simulink library "ddm"  (R2021b)
settings: Solver=VariableStepAuto  StartTime=0.0  StopTime=10.0  RelTol=1e-3
undefined symbols (not defined in the file or in its folder): ENUM_ADASACCSTA_ERROR, ENUM_ADASACCSTA_OFF, ENUM_ADASACCSTA_STANDBY, ENUM_ADASISASTA_OFF, ENUM_ALLOWMOV_ALLOWREADY, ENUM_APS, ENUM_BRKSTA_ERROR, ENUM_BRKSTA_OFF, ENUM_BRKSTA_ON, ENUM_BRKSW_INVALID, ENUM_BRKSW_OFF, ENUM_BRKSW_ON, ENUM_CHGPREACTERRSTA_OBCPRE, ENUM_DCDCFAULTSTA_ANYFAULTLV1, ENUM_DCDCFAULTSTA_ANYFAULTLV2, ENUM_DRIVETRAIN_AWD, ENUM_DRIVETRAIN_FWD, ENUM_DRIVETRAIN_RWD, ENUM_DRSEATSTA_INVALID, ENUM_EDUDRTSTA_NORMAL, ENUM_EPBSTA_APPLIED, ENUM_EPBSTA_RELEASED, ENUM_HVBATTREADYPRE_READY, ENUM_MCUWARN_LV0, ENUM_MCUWARN_LV1, ENUM_MCUWARN_LV2, ENUM_MCUWARN_LV3, ENUM_MCUWARN_NOERROR, ENUM_OBCFAULTSTA_ANYFAULT, ENUM_PAS_R2F2, ENUM_PDFAULT_BATTPDFAIL, ENUM_PDFAULT_DCDCDISABLE, ENUM_PDFAULT_MCUDISABLE, ENUM_PDFAULT_MCUDISCHRG, ENUM_POWERSTA_OFF, ENUM_POWERSTA_ON, ENUM_POWERSTA_READY, ENUM_POWERSTA_STANDBY, ENUM_PRESSINDI_LOW, ENUM_PUFAULT_BATTUPFAIL, ENUM_PUFAULT_DCDCENABLEFAIL, ENUM_PUFAULT_PRECHRGCHKFAIL, ENUM_PUFAULT_SAFETYCHKFAIL, ENUM_PUSTATE_COMPLETED, ENUM_PWRSTASW_OFF, ENUM_PWRSTASW_OFFA, ENUM_PWRSTASW_OFFCHVCHRG, ENUM_PWRSTASW_OFFCLVCHRG, ENUM_PWRSTASW_ON, ENUM_PWRSTASW_ONHVCHRG, ENUM_PWRSTASW_READY, ENUM_PWRSTASW_STANDBY, ENUM_RANGESTA_12IN, ENUM_SHIFTCOMMAND_D, ENUM_SHIFTCOMMAND_N, ENUM_SHIFTCOMMAND_P, ENUM_SHIFTCOMMAND_R, ENUM_VEHMALFUNLV_2ND, ENUM_VEHMALFUNLV_3RD, ENUM_VEHMALFUNLV_4TH ... (+835)
libraries: hcu_lib x750, $bdroot x12, simulink x5
(part 17 of 28)

== system ddm/DDM/DDM/PMM/Comm err/The CAN signal between VCU and CCU2 is incomplete ==
  note: Diagnostics and Fault Handling
  note: Test Detection Criteria
  note: Fail Safe After Decision
  note: Release Condition After Failure Decision
  note: Release Condition During Failure Detection
  note: Fail Safe During Detection
  note: Test Pass Criteria
  task_time_s : Inport
  VPMM_PowerSta_enum : Inport  Port=2
  VPMM_PwrStaSW_enum : Inport  Port=3
  VDDM_C3CCU2CSChk_flg : Inport  Port=4
  VDDM_C3CCU2LCCFS_flg : Inport  Port=5
  No_CAN3_BUS_OFF : Inport  Port=6
  DTC_clear_request : Inport  Port=7
  Constant15 : Constant  Value=KDDM_C3CCU2CSCFSSW_flg
  Constant{3,16,22,24} (4 alike) : Constant  Value=TRUE
  Constant18 : Constant  Value=KDDM_C3CCU2CSPassTO_s
  Constant19 : Constant  Value=KDDM_C3CCU2CSPassTO_s
  Constant{2,21,23,25,27} (5 alike) : Constant  Value=FALSE
  Constant20 : Constant  Value=KDDM_C3CCU2CSDFSSW_flg
  Constant26 : Constant  Value=ENUM_PWRSTASW_OFF
  Constant28 : Constant  Value=ENUM_PWRSTASW_OFF
  Constant4 : Constant  Value=ENUM_POWERSTA_OFF
  Constant40 : Constant  Value=KDDM_C3CCU2CSDTC_cnt
  Constant41 : Constant  Value=KDDM_C3CCU2CSDetTO_s
  Constant46 : Constant  Value=KDDM_C3CCU2CSDetSW_flg
  Constant48 : Constant  Value=KDDM_C3CCU2CSDTC_cnt
  Constant5 : Constant  Value=KDDM_C3CCU2CSPassSW_flg
  DTC_Couter : hcu_lib/Basic_Blocks/DTC_Couter
  DTC_Info : hcu_lib/Basic_Blocks/DTC_Info
  Data Type Conversion1 : DataTypeConversion  OutDataTypeStr=uint8
  Demux : Demux  Commented=on  Outputs=5
  Equal : RelationalOperator  Operator=~=  OutDataTypeStr=boolean  RndMeth=Simplest
  Equal2 : RelationalOperator  Operator=~=  OutDataTypeStr=boolean  RndMeth=Simplest
  Equal3 : RelationalOperator  OutDataTypeStr=boolean  RndMeth=Simplest
  Equal4 : RelationalOperator  Operator===  OutDataTypeStr=boolean  RndMeth=Simplest
  From19 : From  Commented=on  GotoTag=VDDM_C3CCU2CSDFS_flg
  Goto19 : Goto  Commented=on  GotoTag=VDDM_EDriveSysErrVCUErr_flg
  Logical Operator{1,4,6,9} (4 alike) : Logic  Operator=NOT  AllPortsSameDT=off  OutDataTypeStr=boolean
  Logical Operator12 : Logic  AllPortsSameDT=off  OutDataTypeStr=boolean
  Logical Operator15 : Logic  AllPortsSameDT=off  OutDataTypeStr=boolean
  Logical Operator18 : Logic  AllPortsSameDT=off  OutDataTypeStr=boolean
  Logical Operator19 : Logic  Inputs=3  AllPortsSameDT=off  OutDataTypeStr=boolean
  Logical Operator2 : Logic  Inputs=3  AllPortsSameDT=off  OutDataTypeStr=boolean
  Logical Operator21 : Logic  Operator=OR  Inputs=3  AllPortsSameDT=off  OutDataTypeStr=boolean
  Logical Operator3 : Logic  Operator=OR  Inputs=3  AllPortsSameDT=off  OutDataTypeStr=boolean
  Logical Operator5 : Logic  Inputs=3  AllPortsSameDT=off  OutDataTypeStr=boolean
  Logical Operator7 : Logic  Operator=OR  AllPortsSameDT=off  OutDataTypeStr=boolean
  Logical Operator8 : Logic  Operator=OR  AllPortsSameDT=off  OutDataTypeStr=boolean
  Relay : Relay  OnSwitchValue=ONE_INT  OffSwitchValue=ZERO_INT
  SR_Latch1 : Subsystem  mask(SR_Latch){}
      mask help: SR latch function.
  SR_Latch3 : hcu_lib/Basic_Blocks/SR_Latch
  SR_Latch4 : hcu_lib/Basic_Blocks/SR_Latch
  Switch{,1,4..7} (6 alike) : Switch  Criteria=u2 ~= 0
  Switch3 : Switch  Commented=on  Criteria=u2 ~= 0
  Test Detection Criteria : hcu_lib/Basic_Blocks/Test Detection Criteria
  Timer1 : hcu_lib/Basic_Blocks/Timer
  Unit Delay3 : UnitDelay  Commented=on  SampleTime=-1  HasFrameUpgradeWarning=on
  VDDM_C3CCU2CSDTC_raw32 : Outport
  VDDM_C3CCU2CSCFS_flg : Outport  Port=2
  wires:
  Constant15/1 -> Logical Operator18/2
  Constant48/1 -> DTC_Couter/3
  [VDDM_C3CCU2CSDet_flg] -> Logical Operator19/1
  Logical Operator18/1 -> [VDDM_C3CCU2CSCFS_flg]  "VDDM_C3CCU2CSCFS_flg"
  Constant5/1 -> Logical Operator15/2
  Logical Operator3/1 -> Logical Operator15/1
  Constant46/1 -> Logical Operator19/2
  [VDDM_C3CCU2CSCFSRls_flg] -> Logical Operator7/1
  DTC_Couter/1 -> SR_Latch4/1
  [VDDM_C3CCU2CSDTC_cnt] -> Relay/1
  Logical Operator19/1 -> DTC_Couter/1
  [VDDM_C3CCU2CSDFSRls_flg] -> Logical Operator21/1
  Logical Operator21/1 -> SR_Latch3/2
  Logical Operator9/1 -> Logical Operator19/3
  Logical Operator7/1 -> SR_Latch4/2
  SR_Latch3/1 -> Logical Operator12/2
  [VDDM_C3CCU2CSPass_flg] -> Logical Operator3/1
  SR_Latch4/1 -> Logical Operator18/1
  DTC_Couter/2 -> Data Type Conversion1/1
  [VDDM_C3CCU2CSCFS_flg] -> Logical Operator21/2
  Relay/1 -> SR_Latch3/1
  [DTC_clear_request] -> Logical Operator21/3
  Data Type Conversion1/1 -> [VDDM_C3CCU2CSDTC_cnt]  "VDDM_C3CCU2CSDTC_cnt"
  [DTC_clear_request] -> Logical Operator7/2
  [DTC_clear_request] -> Logical Operator9/1
  [DTC_clear_request] -> Logical Operator3/3
  [VDDM_C3CCU2CSCFSRls_flg] -> Logical Operator3/2
  Logical Operator12/1 -> [VDDM_C3CCU2CSDFS_flg]  "VDDM_C3CCU2CSDFS_flg"
  Logical Operator15/1 -> DTC_Couter/2
  Constant20/1 -> Logical Operator12/1
  [VDDM_C3CCU2CSCFS_flg] -> VDDM_C3CCU2CSCFS_flg/1
  Constant2/1 -> Switch1/1
  Switch5/1 -> Switch1/3, [VDDM_xxx_flg]
  Switch1/1 -> Test Detection Criteria/1
  [DTC_clear_request] -> Switch1/2
  [DTC_clear_request] -> DTC_Info/4
  Constant41/1 -> Test Detection Criteria/4
  [VDDM_C3CCU2CSDet_flg] -> DTC_Info/1
  [VDDM_C3CCU2CSPass_flg] -> DTC_Info/2
  [VDDM_C3CCU2CSCFS_flg] -> DTC_Info/3
  DTC_Info/1 -> VDDM_C3CCU2CSDTC_raw32/1  "VDDM_C3CCU2CSDTC_raw32"
  [task_time_s] -> Timer1/3
  [VPMM_PwrStaSW_enum] -> Equal2/1
  [VPMM_PwrStaSW_enum] -> Equal/1
  [VPMM_PowerSta_enum] -> Equal4/1
  From19/1 -> Switch3/2
  Switch4/1 -> [VDDM_C3CCU2CSCFSRls_flg]  "VDDM_C3CCU2CSCFSRls_flg"
  Constant23/1 -> Switch7/3
  Equal4/1 -> Logical Operator8/1
  Logical Operator2/1 -> Switch5/2
  [No_CAN3_BUS_OFF] -> Logical Operator2/1
  [VDDM_C3CCU2LCCFS_flg] -> Logical Operator4/1
  Test Detection Criteria/1 -> [VDDM_C3CCU2CSDet_flg]  "VDDM_C3CCU2CSDet_flg"
  [VDDM_xxx_flg] -> SR_Latch1/2(reset)
  Equal3/1 -> SR_Latch1/1(set)
  Logical Operator4/1 -> Logical Operator5/3
  [VDDM_C3CCU2CSCFS_flg] -> Switch/2
  [VDDM_C3CCU2CSChk_flg] -> Switch6/1
  Logical Operator8/1 -> Switch4/2
  [VDDM_C3CCU2CSPass_flg] -> Switch7/2
  [VDDM_C3CCU2CSChk_flg] -> Switch5/1
  Switch7/1 -> [VDDM_C3CCU2CSDFSRls_flg]  "VDDM_C3CCU2CSDFSRls_flg"
  SR_Latch1/1(latched) -> [VDDM_C3CCU2CSPass_flg]  "VDDM_C3CCU2CSPass_flg"
  Constant25/1 -> Switch4/3
  [DTC_clear_request] -> Logical Operator8/2
  Constant28/1 -> Equal2/2
  Logical Operator6/1 -> Timer1/1
  Timer1/1 -> Equal3/1
  Constant24/1 -> Switch4/1
  [No_CAN3_BUS_OFF] -> Logical Operator5/1
  Equal2/1 -> Logical Operator5/2
  Constant40/1 -> Test Detection Criteria/3
  Logical Operator1/1 -> Logical Operator2/3
  [task_time_s] -> Test Detection Criteria/2
  Switch6/1 -> Timer1/2, Logical Operator6/1
  Switch/1 -> Goto19/1
  Constant16/1 -> Switch6/3
  Constant26/1 -> Equal/2
  Constant3/1 -> Switch/1
  Constant18/1 -> Timer1/4
  Constant27/1 -> Switch5/3
  Demux/1 -> Unit Delay3/1
  Constant4/1 -> Equal4/2
  Equal/1 -> Logical Operator2/2
  Constant19/1 -> Equal3/2
  [VDDM_C3CCU2LCCFS_flg] -> Logical Operator1/1
  Switch3/1 -> Demux/1
  Logical Operator5/1 -> Switch6/2
  Constant21/1 -> Switch/3
  Constant22/1 -> Switch7/1
  DTC_clear_request/1 -> [DTC_clear_request]
  No_CAN3_BUS_OFF/1 -> [No_CAN3_BUS_OFF]
  VDDM_C3CCU2LCCFS_flg/1 -> [VDDM_C3CCU2LCCFS_flg]
  VPMM_PowerSta_enum/1 -> [VPMM_PowerSta_enum]
  VPMM_PwrStaSW_enum/1 -> [VPMM_PwrStaSW_enum]
  VDDM_C3CCU2CSChk_flg/1 -> [VDDM_C3CCU2CSChk_flg]
  task_time_s/1 -> [task_time_s]

== system ddm/DDM/DDM/PMM/Comm err/VCU lost communication with ABM1 ==
  note: Diagnostics and Fault Handling
  note: Fail Safe After Decision
  note: Test Pass Criteria
  note: Test Detection Criteria
  note: Fail Safe During Detection
  note: Release Condition After Failure Decision
  note: Release Condition During Failure Detection
  task_time_s : Inport
  VPMM_PowerSta_enum : Inport  Port=2
  VPMM_PwrStaSW_enum : Inport  Port=3
  VDDM_C1ABM1LCChk_flg : Inport  Port=4
  No_CAN1_BUS_OFF : Inport  Port=5
  DTC_clear_request : Inport  Port=6
  Constant15 : Constant  Value=KDDM_C1ABM1LCCFSSW_flg
  Constant16 : Constant  Value=TRUE
  Constant18 : Constant  Value=KDDM_C1ABM1LCPassTO_s
  Constant19 : Constant  Value=KDDM_C1ABM1LCPassTO_s
  Constant{2,21,25,27} (4 alike) : Constant  Value=FALSE
  Constant20 : Constant  Value=KDDM_C1ABM1LCDFSSW_flg
  Constant24 : Constant  Value=TRUE
  Constant26 : Constant  Value=ENUM_PWRSTASW_OFF
  Constant28 : Constant  Value=ENUM_PWRSTASW_OFF
  Constant3 : Constant  Value=TRUE
  Constant4 : Constant  Value=ENUM_POWERSTA_OFF
  Constant40 : Constant  Value=KDDM_C1ABM1LCDTC_cnt
  Constant41 : Constant  Value=KDDM_C1ABM1LCDetTO_s
  Constant46 : Constant  Value=KDDM_C1ABM1LCDetSW_flg
  Constant48 : Constant  Value=KDDM_C1ABM1LCDTC_cnt
  Constant5 : Constant  Value=KDDM_C1ABM1LCPassSW_flg
  DTC_Couter : hcu_lib/Basic_Blocks/DTC_Couter
  DTC_Info : hcu_lib/Basic_Blocks/DTC_Info
  Data Type Conversion1 : DataTypeConversion  OutDataTypeStr=uint8
  Equal : RelationalOperator  Operator=~=  OutDataTypeStr=boolean  RndMeth=Simplest
  Equal2 : RelationalOperator  Operator=~=  OutDataTypeStr=boolean  RndMeth=Simplest
  Equal3 : RelationalOperator  OutDataTypeStr=boolean  RndMeth=Simplest
  Equal4 : RelationalOperator  Operator===  OutDataTypeStr=boolean  RndMeth=Simplest
  Logical Operator1 : Logic  Operator=NOT  AllPortsSameDT=off  OutDataTypeStr=boolean
  Logical Operator{2,5,12,15,18} (5 alike) : Logic  AllPortsSameDT=off  OutDataTypeStr=boolean
  Logical Operator19 : Logic  Inputs=3  AllPortsSameDT=off  OutDataTypeStr=boolean
  Logical Operator3 : Logic  Operator=OR  Inputs=3  AllPortsSameDT=off  OutDataTypeStr=boolean
  Logical Operator4 : Logic  Operator=OR  AllPortsSameDT=off  OutDataTypeStr=boolean
  Logical Operator6 : Logic  Operator=NOT  AllPortsSameDT=off  OutDataTypeStr=boolean
  Logical Operator7 : Logic  Operator=OR  AllPortsSameDT=off  OutDataTypeStr=boolean
  Logical Operator8 : Logic  Operator=OR  AllPortsSameDT=off  OutDataTypeStr=boolean
  Relay : Relay  OnSwitchValue=ONE_INT  OffSwitchValue=ZERO_INT
  SR_Latch1 : Subsystem  mask(SR_Latch){}
      mask help: SR latch function.
  SR_Latch3 : hcu_lib/Basic_Blocks/SR_Latch
  SR_Latch4 : hcu_lib/Basic_Blocks/SR_Latch
  Switch{,1,4..6} (5 alike) : Switch  Criteria=u2 ~= 0
  Test Detection Criteria : hcu_lib/Basic_Blocks/Test Detection Criteria
  Timer1 : hcu_lib/Basic_Blocks/Timer
  VDDM_C1ABM1LCDTC_raw32 : Outport
  VDDM_C1ABM1LCCFS_flg : Outport  Port=2
  LC_EDriveSysErr_VCUErr_flg : Outport  Port=3
  wires:
  [DTC_clear_request] -> Logical Operator7/2
  [VDDM_C1ABM1LCPass_flg] -> Logical Operator3/1
  Logical Operator12/1 -> [VDDM_C1ABM1LCDFS_flg]  "VDDM_C1ABM1LCDFS_flg"
  Logical Operator1/1 -> Logical Operator19/3
  SR_Latch4/1 -> Logical Operator18/1
  Logical Operator4/1 -> SR_Latch4/2
  [DTC_clear_request] -> Logical Operator4/2
  [DTC_clear_request] -> Logical Operator1/1
  Logical Operator18/1 -> [VDDM_C1ABM1LCCFS_flg]  "VDDM_C1ABM1LCCFS_flg"
  [VDDM_C1ABM1LCCFS_flg] -> Logical Operator7/1
  [VDDM_C1ABM1LCCFSRls_flg] -> Logical Operator3/2
  Logical Operator15/1 -> DTC_Couter/2
  Constant15/1 -> Logical Operator18/2
  DTC_Couter/2 -> Data Type Conversion1/1
  [VDDM_C1ABM1LCCFSRls_flg] -> Logical Operator4/1
  DTC_Couter/1 -> SR_Latch4/1
  [VDDM_C1ABM1LCDet_flg] -> Logical Operator19/1
  Logical Operator3/1 -> Logical Operator15/1
  Logical Operator7/1 -> SR_Latch3/2
  Constant46/1 -> Logical Operator19/2
  [DTC_clear_request] -> Logical Operator3/3
  SR_Latch3/1 -> Logical Operator12/2
  [VDDM_C1ABM1LCDTC_cnt] -> Relay/1
  Relay/1 -> SR_Latch3/1
  Logical Operator19/1 -> DTC_Couter/1
  Constant48/1 -> DTC_Couter/3
  Constant20/1 -> Logical Operator12/1
  Data Type Conversion1/1 -> [VDDM_C1ABM1LCDTC_cnt]  "VDDM_C1ABM1LCDTC_cnt"
  Constant5/1 -> Logical Operator15/2
  Constant2/1 -> Switch1/1
  Switch5/1 -> Switch1/3, [VDDM_xxx_flg]
  Switch1/1 -> Test Detection Criteria/1
  [DTC_clear_request] -> Switch1/2
  [DTC_clear_request] -> DTC_Info/4
  Constant41/1 -> Test Detection Criteria/4
  [VDDM_C1ABM1LCPass_flg] -> DTC_Info/2
  [VDDM_C1ABM1LCDet_flg] -> DTC_Info/1
  [VDDM_C1ABM1LCCFS_flg] -> VDDM_C1ABM1LCCFS_flg/1, DTC_Info/3
  DTC_Info/1 -> VDDM_C1ABM1LCDTC_raw32/1  "VDDM_C1ABM1LCDTC_raw32"
  [task_time_s] -> Timer1/3
  [VPMM_PwrStaSW_enum] -> Equal2/1
  [VPMM_PwrStaSW_enum] -> Equal/1
  [VPMM_PowerSta_enum] -> Equal4/1
  [EDriveSysErr_VCUErr_flg] -> LC_EDriveSysErr_VCUErr_flg/1
  Constant4/1 -> Equal4/2
  Constant18/1 -> Timer1/4
  Equal3/1 -> SR_Latch1/1(set)
  Switch6/1 -> Timer1/2, Logical Operator6/1
  SR_Latch1/1(latched) -> [VDDM_C1ABM1LCPass_flg]  "VDDM_C1ABM1LCPass_flg"
  Constant28/1 -> Equal2/2
  [VDDM_C1ABM1LCChk_flg] -> Switch5/1
  Logical Operator8/1 -> Switch4/2
  [VDDM_C1ABM1LCChk_flg] -> Switch6/1
  Switch4/1 -> [VDDM_C1ABM1LCCFSRls_flg]  "VDDM_C1ABM1LCCFSRls_flg"
  Constant25/1 -> Switch4/3
  Equal2/1 -> Logical Operator5/2
  [VDDM_C1ABM1LCCFS_flg] -> Switch/2
  Constant21/1 -> Switch/3
  Constant40/1 -> Test Detection Criteria/3
  [VDDM_xxx_flg] -> SR_Latch1/2(reset)
  [No_CAN1_BUS_OFF] -> Logical Operator5/1
  Switch/1 -> [EDriveSysErr_VCUErr_flg]
  Logical Operator5/1 -> Switch6/2
  Logical Operator2/1 -> Switch5/2
  Constant24/1 -> Switch4/1
  Constant26/1 -> Equal/2
  [DTC_clear_request] -> Logical Operator8/2
  [No_CAN1_BUS_OFF] -> Logical Operator2/1
  Constant27/1 -> Switch5/3
  Timer1/1 -> Equal3/1
  Equal4/1 -> Logical Operator8/1
  Equal/1 -> Logical Operator2/2
  [task_time_s] -> Test Detection Criteria/2
  Logical Operator6/1 -> Timer1/1
  Constant16/1 -> Switch6/3
  Constant19/1 -> Equal3/2
  Test Detection Criteria/1 -> [VDDM_C1ABM1LCDet_flg]  "VDDM_C1ABM1LCDet_flg"
  Constant3/1 -> Switch/1
  No_CAN1_BUS_OFF/1 -> [No_CAN1_BUS_OFF]
  DTC_clear_request/1 -> [DTC_clear_request]
  task_time_s/1 -> [task_time_s]
  VDDM_C1ABM1LCChk_flg/1 -> [VDDM_C1ABM1LCChk_flg]
  VPMM_PwrStaSW_enum/1 -> [VPMM_PwrStaSW_enum]
  VPMM_PowerSta_enum/1 -> [VPMM_PowerSta_enum]

== system ddm/DDM/DDM/PMM/Comm err/VCU lost communication with BMS1 ==
  note: Diagnostics and Fault Handling
  note: Test Detection Criteria
  note: Test Pass Criteria
  note: Release Condition During Failure Detection
  note: Fail Safe During Detection
  note: Fail Safe After Decision
  note: Release Condition After Failure Decision
  task_time_s : Inport
  VPMM_PowerSta_enum : Inport  Port=2
  VPMM_PwrStaSW_enum : Inport  Port=3
  VDDM_C3BMS1LCChk_flg : Inport  Port=4
  No_CAN3_BUS_OFF : Inport  Port=5
  DTC_clear_request : Inport  Port=6
  Constant15 : Constant  Value=KDDM_C3BMS1LCCFSSW_flg
  Constant{3,16,22,24} (4 alike) : Constant  Value=TRUE
  Constant18 : Constant  Value=KDDM_C3BMS1LCPassTO_s
  Constant19 : Constant  Value=KDDM_C3BMS1LCPassTO_s
  Constant{2,21,23,25,27} (5 alike) : Constant  Value=FALSE
  Constant20 : Constant  Value=KDDM_C3BMS1LCDFSSW_flg
  Constant26 : Constant  Value=ENUM_PWRSTASW_OFF
  Constant28 : Constant  Value=ENUM_PWRSTASW_OFF
  Constant4 : Constant  Value=ENUM_POWERSTA_OFF
  Constant40 : Constant  Value=KDDM_C3BMS1LCDTC_cnt
  Constant41 : Constant  Value=KDDM_C3BMS1LCDetTO_s
  Constant46 : Constant  Value=KDDM_C3BMS1LCDetSW_flg
  Constant48 : Constant  Value=KDDM_C3BMS1LCDTC_cnt
  Constant5 : Constant  Value=KDDM_C3BMS1LCPassSW_flg
  DTC_Couter : hcu_lib/Basic_Blocks/DTC_Couter
  DTC_Info : hcu_lib/Basic_Blocks/DTC_Info
  Data Type Conversion1 : DataTypeConversion  OutDataTypeStr=uint8
  Demux : Demux  Commented=on  Outputs=5
  Equal : RelationalOperator  Operator=~=  OutDataTypeStr=boolean  RndMeth=Simplest
  Equal2 : RelationalOperator  Operator=~=  OutDataTypeStr=boolean  RndMeth=Simplest
  Equal3 : RelationalOperator  OutDataTypeStr=boolean  RndMeth=Simplest
  Equal4 : RelationalOperator  Operator===  OutDataTypeStr=boolean  RndMeth=Simplest
  From19 : From  Commented=on  GotoTag=VDDM_C3BMS1LCDFS_flg
  Goto19 : Goto  Commented=on  GotoTag=VDDM_EDriveSysErrVCUErr_flg
  Logical Operator1 : Logic  Operator=NOT  AllPortsSameDT=off  OutDataTypeStr=boolean
  Logical Operator{2,5,12,15,18} (5 alike) : Logic  AllPortsSameDT=off  OutDataTypeStr=boolean
  Logical Operator19 : Logic  Inputs=3  AllPortsSameDT=off  OutDataTypeStr=boolean
  Logical Operator21 : Logic  Operator=OR  Inputs=3  AllPortsSameDT=off  OutDataTypeStr=boolean
  Logical Operator3 : Logic  Operator=OR  Inputs=3  AllPortsSameDT=off  OutDataTypeStr=boolean
  Logical Operator4 : Logic  Operator=OR  AllPortsSameDT=off  OutDataTypeStr=boolean
  Logical Operator6 : Logic  Operator=NOT  AllPortsSameDT=off  OutDataTypeStr=boolean
  Logical Operator8 : Logic  Operator=OR  AllPortsSameDT=off  OutDataTypeStr=boolean
  Relay : Relay  OnSwitchValue=ONE_INT  OffSwitchValue=ZERO_INT
  SR_Latch1 : Subsystem  mask(SR_Latch){}
      mask help: SR latch function.
  SR_Latch3 : hcu_lib/Basic_Blocks/SR_Latch
  SR_Latch4 : hcu_lib/Basic_Blocks/SR_Latch
  Switch{,1,4..7} (6 alike) : Switch  Criteria=u2 ~= 0
  Switch3 : Switch  Commented=on  Criteria=u2 ~= 0
  Test Detection Criteria : hcu_lib/Basic_Blocks/Test Detection Criteria
  Timer1 : hcu_lib/Basic_Blocks/Timer
  Unit Delay3 : UnitDelay  Commented=on  SampleTime=-1  HasFrameUpgradeWarning=on
  VDDM_C3BMS1LCDTC_raw32 : Outport
  VDDM_C3BMS1LCCFS_flg : Outport  Port=2
  wires:
  Logical Operator21/1 -> SR_Latch3/2
  Constant5/1 -> Logical Operator15/2
  Relay/1 -> SR_Latch3/1
  Constant48/1 -> DTC_Couter/3
  Constant20/1 -> Logical Operator12/1
  Logical Operator15/1 -> DTC_Couter/2
  [DTC_clear_request] -> Logical Operator1/1
  [DTC_clear_request] -> Logical Operator21/3
  [DTC_clear_request] -> Logical Operator3/3
  [DTC_clear_request] -> Logical Operator4/2
  Constant46/1 -> Logical Operator19/2
  DTC_Couter/2 -> Data Type Conversion1/1
  Logical Operator3/1 -> Logical Operator15/1
  Logical Operator1/1 -> Logical Operator19/3
  [VDDM_C3BMS1LCCFSRls_flg] -> Logical Operator4/1
  Data Type Conversion1/1 -> [VDDM_C3BMS1LCDTC_cnt]  "VDDM_C3BMS1LCDTC_cnt"
  Logical Operator4/1 -> SR_Latch4/2
  [VDDM_C3BMS1LCCFS_flg] -> Logical Operator21/2
  Logical Operator18/1 -> [VDDM_C3BMS1LCCFS_flg]  "VDDM_C3BMS1LCCFS_flg"
  DTC_Couter/1 -> SR_Latch4/1
  [VDDM_C3BMS1LCCFSRls_flg] -> Logical Operator3/2
  Logical Operator19/1 -> DTC_Couter/1
  SR_Latch4/1 -> Logical Operator18/1
  [VDDM_C3BMS1LCPass_flg] -> Logical Operator3/1
  SR_Latch3/1 -> Logical Operator12/2
  [VDDM_C3BMS1LCDTC_cnt] -> Relay/1
  [VDDM_C3BMS1LCDet_flg] -> Logical Operator19/1
  Constant15/1 -> Logical Operator18/2
  Logical Operator12/1 -> [VDDM_C3BMS1LCDFS_flg]  "VDDM_C3BMS1LCDFS_flg"
  [VDDM_C3BMS1LCDFSRls_flg] -> Logical Operator21/1
  Constant2/1 -> Switch1/1
  Switch5/1 -> Switch1/3, [VDDM_xxx_flg]
  Switch1/1 -> Test Detection Criteria/1
  [DTC_clear_request] -> Switch1/2
  [DTC_clear_request] -> DTC_Info/4
  Constant41/1 -> Test Detection Criteria/4
  [VDDM_C3BMS1LCPass_flg] -> DTC_Info/2
  [VDDM_C3BMS1LCDet_flg] -> DTC_Info/1
  DTC_Info/1 -> VDDM_C3BMS1LCDTC_raw32/1  "VDDM_C3BMS1LCDTC_raw32"
  [task_time_s] -> Timer1/3
  [VPMM_PwrStaSW_enum] -> Equal2/1
  [VPMM_PwrStaSW_enum] -> Equal/1
  [VPMM_PowerSta_enum] -> Equal4/1
  [DTC_clear_request] -> Logical Operator8/2
  Switch4/1 -> [VDDM_C3BMS1LCCFSRls_flg]  "VDDM_C3BMS1LCCFSRls_flg"
  Constant25/1 -> Switch4/3
  Equal4/1 -> Logical Operator8/1
  SR_Latch1/1(latched) -> [VDDM_C3BMS1LCPass_flg]  "VDDM_C3BMS1LCPass_flg"
  Switch7/1 -> [VDDM_C3BMS1LCDFSRls_flg]  "VDDM_C3BMS1LCDFSRls_flg"
  [VDDM_C3BMS1LCChk_flg] -> Switch5/1
  Logical Operator8/1 -> Switch4/2
  [VDDM_C3BMS1LCChk_flg] -> Switch6/1
  Equal3/1 -> SR_Latch1/1(set)
  Logical Operator2/1 -> Switch5/2
  From19/1 -> Switch3/2
  Test Detection Criteria/1 -> [VDDM_C3BMS1LCDet_flg]  "VDDM_C3BMS1LCDet_flg"
  [No_CAN3_BUS_OFF] -> Logical Operator2/1
  Constant23/1 -> Switch7/3
  Constant27/1 -> Switch5/3
  Constant18/1 -> Timer1/4
  Constant3/1 -> Switch/1
  Timer1/1 -> Equal3/1
  Switch6/1 -> Timer1/2, Logical Operator6/1
  Constant16/1 -> Switch6/3
  Switch/1 -> Goto19/1
  [VDDM_xxx_flg] -> SR_Latch1/2(reset)
  Constant26/1 -> Equal/2
  Equal2/1 -> Logical Operator5/2
  Constant40/1 -> Test Detection Criteria/3
  Constant24/1 -> Switch4/1
  [VDDM_C3BMS1LCPass_flg] -> Switch7/2
  [No_CAN3_BUS_OFF] -> Logical Operator5/1
  Logical Operator6/1 -> Timer1/1
  [VDDM_C3BMS1LCCFS_flg] -> Switch/2
  Constant22/1 -> Switch7/1
  Constant28/1 -> Equal2/2
  Constant21/1 -> Switch/3
  Logical Operator5/1 -> Switch6/2
  Switch3/1 -> Demux/1
  Constant4/1 -> Equal4/2
  Equal/1 -> Logical Operator2/2
  Constant19/1 -> Equal3/2
  [task_time_s] -> Test Detection Criteria/2
  Demux/1 -> Unit Delay3/1
  DTC_clear_request/1 -> [DTC_clear_request]
  No_CAN3_BUS_OFF/1 -> [No_CAN3_BUS_OFF]
  VPMM_PowerSta_enum/1 -> [VPMM_PowerSta_enum]
  VPMM_PwrStaSW_enum/1 -> [VPMM_PwrStaSW_enum]
  VDDM_C3BMS1LCChk_flg/1 -> [VDDM_C3BMS1LCChk_flg]
  task_time_s/1 -> [task_time_s]
  [VDDM_C3BMS1LCCFS_flg] -> VDDM_C3BMS1LCCFS_flg/1, DTC_Info/3

== system ddm/DDM/DDM/PMM/Comm err/VCU lost communication with BMS6 ==
  note: Diagnostics and Fault Handling
  note: Fail Safe During Detection
  note: Test Pass Criteria
  note: Release Condition During Detection
  note: Test Detection Criteria
  note: Fail Safe After Decision
  note: Release Condition After Decision
  task_time_s : Inport
  VPMM_PowerSta_enum : Inport  Port=2
  VPMM_PwrStaSW_enum : Inport  Port=3
  VDDM_C3BMS6LCChk_flg : Inport  Port=4
  No_CAN3_BUS_OFF : Inport  Port=5
  DTC_clear_request : Inport  Port=6
  Constant15 : Constant  Value=KDDM_C3BMS6LCCFSSW_flg
  Constant{3,16,22,24} (4 alike) : Constant  Value=TRUE
  Constant18 : Constant  Value=KDDM_C3BMS6LCPassTO_s
  Constant19 : Constant  Value=KDDM_C3BMS6LCPassTO_s
  Constant{2,21,23,25,28} (5 alike) : Constant  Value=FALSE
  Constant20 : Constant  Value=KDDM_C3BMS6LCDFSSW_flg
  Constant26 : Constant  Value=ENUM_PWRSTASW_OFF
  Constant29 : Constant  Value=ENUM_PWRSTASW_OFF
  Constant4 : Constant  Value=ENUM_POWERSTA_OFF
  Constant40 : Constant  Value=KDDM_C3BMS6LCDTC_cnt
  Constant41 : Constant  Value=KDDM_C3BMS6LCDetTO_s
  Constant46 : Constant  Value=KDDM_C3BMS6LCDetSW_flg
  Constant48 : Constant  Value=KDDM_C3BMS6LCDTC_cnt
  Constant5 : Constant  Value=KDDM_C3BMS6LCPassSW_flg
  DTC_Couter : hcu_lib/Basic_Blocks/DTC_Couter
  DTC_Info : hcu_lib/Basic_Blocks/DTC_Info
  Data Type Conversion1 : DataTypeConversion  OutDataTypeStr=uint8
  Demux : Demux  Commented=on  Outputs=5
  Equal : RelationalOperator  Operator=~=  OutDataTypeStr=boolean  RndMeth=Simplest
  Equal2 : RelationalOperator  Operator=~=  OutDataTypeStr=boolean  RndMeth=Simplest
  Equal3 : RelationalOperator  OutDataTypeStr=boolean  RndMeth=Simplest
  Equal4 : RelationalOperator  Operator===  OutDataTypeStr=boolean  RndMeth=Simplest
  From13 : From  Commented=on  GotoTag=VDDM_C3BMS6LCDFS_flg
  Goto16 : Goto  Commented=on  GotoTag=VDDM_EDriveSysErrVCUErr_flg
  Logical Operator1 : Logic  Operator=OR  AllPortsSameDT=off  OutDataTypeStr=boolean
  Logical Operator{2,4,12,15,18} (5 alike) : Logic  AllPortsSameDT=off  OutDataTypeStr=boolean
  Logical Operator19 : Logic  Inputs=3  AllPortsSameDT=off  OutDataTypeStr=boolean
  Logical Operator21 : Logic  Operator=OR  Inputs=3  AllPortsSameDT=off  OutDataTypeStr=boolean
  Logical Operator3 : Logic  Operator=OR  Inputs=3  AllPortsSameDT=off  OutDataTypeStr=boolean
  Logical Operator5 : Logic  Operator=NOT  AllPortsSameDT=off  OutDataTypeStr=boolean
  Logical Operator6 : Logic  Operator=NOT  AllPortsSameDT=off  OutDataTypeStr=boolean
  Logical Operator8 : Logic  Operator=OR  AllPortsSameDT=off  OutDataTypeStr=boolean
  Relay : Relay  OnSwitchValue=ONE_INT  OffSwitchValue=ZERO_INT
  SR_Latch1 : Subsystem  mask(SR_Latch){}
      mask help: SR latch function.
  SR_Latch3 : hcu_lib/Basic_Blocks/SR_Latch
  SR_Latch4 : hcu_lib/Basic_Blocks/SR_Latch
  Switch{,1,4..7} (6 alike) : Switch  Criteria=u2 ~= 0
  Switch3 : Switch  Commented=on  Criteria=u2 ~= 0
  Test Detection Criteria : hcu_lib/Basic_Blocks/Test Detection Criteria
  Timer1 : hcu_lib/Basic_Blocks/Timer
  Unit Delay3 : UnitDelay  Commented=on  SampleTime=-1  HasFrameUpgradeWarning=on
  VDDM_C3BMS6LCDTC_raw32 : Outport
  VDDM_C3BMS6LCCFS_flg : Outport  Port=2
  wires:
  Constant5/1 -> Logical Operator15/2
  Logical Operator21/1 -> SR_Latch3/2
  Logical Operator3/1 -> Logical Operator15/1
  [VDDM_C3BMS6LCDTC_cnt] -> Relay/1
  Constant46/1 -> Logical Operator19/2
  Logical Operator5/1 -> Logical Operator19/3
  [VDDM_C3BMS6LCCFSRls_flg] -> Logical Operator1/1
  Relay/1 -> SR_Latch3/1
  Logical Operator12/1 -> [VDDM_C3BMS6LCDFS_flg]  "VDDM_C3BMS6LCDFS_flg"
  Data Type Conversion1/1 -> [VDDM_C3BMS6LCDTC_cnt]  "VDDM_C3BMS6LCDTC_cnt"
  [DTC_clear_request] -> Logical Operator5/1
  [DTC_clear_request] -> Logical Operator3/3
  Constant20/1 -> Logical Operator12/1
  Constant48/1 -> DTC_Couter/3
  [VDDM_C3BMS6LCDFSRls_flg] -> Logical Operator21/1
  DTC_Couter/1 -> SR_Latch4/1
  [VDDM_C3BMS6LCDet_flg] -> Logical Operator19/1
  DTC_Couter/2 -> Data Type Conversion1/1
  Logical Operator15/1 -> DTC_Couter/2
  Logical Operator18/1 -> [VDDM_C3BMS6LCCFS_flg]  "VDDM_C3BMS6LCCFS_flg"
  SR_Latch3/1 -> Logical Operator12/2
  [DTC_clear_request] -> Logical Operator21/3
  Logical Operator1/1 -> SR_Latch4/2
  [VDDM_C3BMS6LCPass_flg] -> Logical Operator3/1
  Constant15/1 -> Logical Operator18/2
  [VDDM_C3BMS6LCCFS_flg] -> Logical Operator21/2
  SR_Latch4/1 -> Logical Operator18/1
  [DTC_clear_request] -> Logical Operator1/2
  [VDDM_C3BMS6LCCFSRls_flg] -> Logical Operator3/2
  Logical Operator19/1 -> DTC_Couter/1
  Constant2/1 -> Switch1/1
  Switch5/1 -> Switch1/3, [VDDM_xxx_flg]
  Switch1/1 -> Test Detection Criteria/1
  [DTC_clear_request] -> Switch1/2
  [DTC_clear_request] -> DTC_Info/4
  Constant41/1 -> Test Detection Criteria/4
  [VDDM_C3BMS6LCDet_flg] -> DTC_Info/1
  DTC_Info/1 -> VDDM_C3BMS6LCDTC_raw32/1  "VDDM_C3BMS6LCDTC_raw32"
  [VDDM_C3BMS6LCPass_flg] -> DTC_Info/2
  [task_time_s] -> Timer1/3
  [VPMM_PwrStaSW_enum] -> Equal2/1
  [VPMM_PwrStaSW_enum] -> Equal/1
  [VPMM_PowerSta_enum] -> Equal4/1
  No_CAN3_BUS_OFF/1 -> [No_CAN3_BUS_OFF]
  DTC_clear_request/1 -> [DTC_clear_request]
  [VDDM_xxx_flg] -> SR_Latch1/2(reset)
  [VDDM_C3BMS6LCChk_flg] -> Switch6/1
  Switch6/1 -> Timer1/2, Logical Operator6/1
  Demux/1 -> Unit Delay3/1
  [No_CAN3_BUS_OFF] -> Logical Operator4/1
  Constant19/1 -> Equal3/2
  Switch3/1 -> Demux/1
  Equal3/1 -> SR_Latch1/1(set)
  Constant4/1 -> Equal4/2
  Timer1/1 -> Equal3/1
  Constant18/1 -> Timer1/4
  Constant22/1 -> Switch7/1
  Switch/1 -> Goto16/1
  Logical Operator6/1 -> Timer1/1
  Constant26/1 -> Equal/2
  Constant25/1 -> Switch4/3
  Constant24/1 -> Switch4/1
  Constant28/1 -> Switch5/3
  Constant23/1 -> Switch7/3
  Logical Operator4/1 -> Switch6/2
  Constant40/1 -> Test Detection Criteria/3
  [VDDM_C3BMS6LCPass_flg] -> Switch7/2
  Equal4/1 -> Logical Operator8/1
  Constant29/1 -> Equal2/2
  Switch4/1 -> [VDDM_C3BMS6LCCFSRls_flg]  "VDDM_C3BMS6LCCFSRls_flg"
  Logical Operator2/1 -> Switch5/2
  [No_CAN3_BUS_OFF] -> Logical Operator2/1
  [DTC_clear_request] -> Logical Operator8/2
  SR_Latch1/1(latched) -> [VDDM_C3BMS6LCPass_flg]  "VDDM_C3BMS6LCPass_flg"
  From13/1 -> Switch3/2
  Constant16/1 -> Switch6/3
  Logical Operator8/1 -> Switch4/2
  Equal2/1 -> Logical Operator4/2
  Switch7/1 -> [VDDM_C3BMS6LCDFSRls_flg]  "VDDM_C3BMS6LCDFSRls_flg"
  Constant21/1 -> Switch/3
  Equal/1 -> Logical Operator2/2
  [VDDM_C3BMS6LCCFS_flg] -> Switch/2
  Test Detection Criteria/1 -> [VDDM_C3BMS6LCDet_flg]  "VDDM_C3BMS6LCDet_flg"
  [task_time_s] -> Test Detection Criteria/2
  Constant3/1 -> Switch/1
  [VDDM_C3BMS6LCChk_flg] -> Switch5/1
  [VDDM_C3BMS6LCCFS_flg] -> VDDM_C3BMS6LCCFS_flg/1, DTC_Info/3
  task_time_s/1 -> [task_time_s]
  VDDM_C3BMS6LCChk_flg/1 -> [VDDM_C3BMS6LCChk_flg]
  VPMM_PwrStaSW_enum/1 -> [VPMM_PwrStaSW_enum]
  VPMM_PowerSta_enum/1 -> [VPMM_PowerSta_enum]

== system ddm/DDM/DDM/PMM/Comm err/VCU lost communication with CCU1 ==
  note: Diagnostics and Fault Handling
  note: Release Condition During Failure Detection
  note: Release Condition After Failure Decision
  note: Fail Safe After Decision
  note: Test Detection Criteria
  note: Test Pass Criteria
  note: Fail Safe During Detection
  task_time_s : Inport
  VPMM_PowerSta_enum : Inport  Port=2
  VPMM_PwrStaSW_enum : Inport  Port=3
  VDDM_C3CCU1LCChk_flg : Inport  Port=4
  No_CAN3_BUS_OFF : Inport  Port=5
  DTC_clear_request : Inport  Port=6
  Constant15 : Constant  Value=KDDM_C3CCU1LCCFSSW_flg
  Constant{3,16,22,24} (4 alike) : Constant  Value=TRUE
  Constant18 : Constant  Value=KDDM_C3CCU1LCPassTO_s
  Constant19 : Constant  Value=KDDM_C3CCU1LCPassTO_s
  Constant{2,21,23,25,27} (5 alike) : Constant  Value=FALSE
  Constant20 : Constant  Value=KDDM_C3CCU1LCDFSSW_flg
  Constant26 : Constant  Value=ENUM_PWRSTASW_OFF
  Constant28 : Constant  Value=ENUM_PWRSTASW_OFF
  Constant4 : Constant  Value=ENUM_POWERSTA_OFF
  Constant40 : Constant  Value=KDDM_C3CCU1LCDTC_cnt
  Constant41 : Constant  Value=KDDM_C3CCU1LCDetTO_s
  Constant46 : Constant  Value=KDDM_C3CCU1LCDetSW_flg
  Constant48 : Constant  Value=KDDM_C3CCU1LCDTC_cnt
  Constant5 : Constant  Value=KDDM_C3CCU1LCPassSW_flg
  DTC_Couter : hcu_lib/Basic_Blocks/DTC_Couter
  DTC_Info : hcu_lib/Basic_Blocks/DTC_Info
  Data Type Conversion1 : DataTypeConversion  OutDataTypeStr=uint8
  Demux : Demux  Commented=on  Outputs=5
  Equal : RelationalOperator  Operator=~=  OutDataTypeStr=boolean  RndMeth=Simplest
  Equal2 : RelationalOperator  Operator=~=  OutDataTypeStr=boolean  RndMeth=Simplest
  Equal3 : RelationalOperator  OutDataTypeStr=boolean  RndMeth=Simplest
  Equal4 : RelationalOperator  Operator===  OutDataTypeStr=boolean  RndMeth=Simplest
  From19 : From  Commented=on  GotoTag=VDDM_C3CCU1LCDFS_flg
  Goto19 : Goto  Commented=on  GotoTag=VDDM_EDriveSysErrVCUErr_flg
  Logical Operator1 : Logic  Operator=OR  AllPortsSameDT=off  OutDataTypeStr=boolean
  Logical Operator{2,5,12,15,18} (5 alike) : Logic  AllPortsSameDT=off  OutDataTypeStr=boolean
  Logical Operator19 : Logic  Inputs=3  AllPortsSameDT=off  OutDataTypeStr=boolean
  Logical Operator21 : Logic  Operator=OR  Inputs=3  AllPortsSameDT=off  OutDataTypeStr=boolean
  Logical Operator3 : Logic  Operator=OR  Inputs=3  AllPortsSameDT=off  OutDataTypeStr=boolean
  Logical Operator4 : Logic  Operator=NOT  AllPortsSameDT=off  OutDataTypeStr=boolean
  Logical Operator6 : Logic  Operator=NOT  AllPortsSameDT=off  OutDataTypeStr=boolean
  Logical Operator8 : Logic  Operator=OR  AllPortsSameDT=off  OutDataTypeStr=boolean
  Relay : Relay  OnSwitchValue=ONE_INT  OffSwitchValue=ZERO_INT
  SR_Latch1 : Subsystem  mask(SR_Latch){}
      mask help: SR latch function.
  SR_Latch3 : hcu_lib/Basic_Blocks/SR_Latch
  SR_Latch4 : hcu_lib/Basic_Blocks/SR_Latch
  Switch{,1,4..7} (6 alike) : Switch  Criteria=u2 ~= 0
  Switch3 : Switch  Commented=on  Criteria=u2 ~= 0
  Test Detection Criteria : hcu_lib/Basic_Blocks/Test Detection Criteria
  Timer1 : hcu_lib/Basic_Blocks/Timer
  Unit Delay3 : UnitDelay  Commented=on  SampleTime=-1  HasFrameUpgradeWarning=on
  VDDM_C3CCU1LCDTC_raw32 : Outport
  VDDM_C3CCU1LCCFS_flg : Outport  Port=2
  wires:
  [DTC_clear_request] -> Logical Operator21/3
  [VDDM_C3CCU1LCPass_flg] -> Logical Operator3/1
  Logical Operator21/1 -> SR_Latch3/2
  Logical Operator4/1 -> Logical Operator19/3
  [VDDM_C3CCU1LCDTC_cnt] -> Relay/1
  Constant48/1 -> DTC_Couter/3
  [DTC_clear_request] -> Logical Operator4/1
  Logical Operator3/1 -> Logical Operator15/1
  DTC_Couter/1 -> SR_Latch4/1
  [DTC_clear_request] -> Logical Operator1/2
  Logical Operator19/1 -> DTC_Couter/1
  [DTC_clear_request] -> Logical Operator3/3
  Data Type Conversion1/1 -> [VDDM_C3CCU1LCDTC_cnt]  "VDDM_C3CCU1LCDTC_cnt"
  SR_Latch4/1 -> Logical Operator18/1
  Logical Operator18/1 -> [VDDM_C3CCU1LCCFS_flg]  "VDDM_C3CCU1LCCFS_flg"
  SR_Latch3/1 -> Logical Operator12/2
  [VDDM_C3CCU1LCCFSRls_flg] -> Logical Operator1/1
  Logical Operator15/1 -> DTC_Couter/2
  [VDDM_C3CCU1LCDet_flg] -> Logical Operator19/1
  [VDDM_C3CCU1LCCFS_flg] -> Logical Operator21/2
  Constant15/1 -> Logical Operator18/2
  Constant20/1 -> Logical Operator12/1
  [VDDM_C3CCU1LCDFSRls_flg] -> Logical Operator21/1
  [VDDM_C3CCU1LCCFSRls_flg] -> Logical Operator3/2
  Constant46/1 -> Logical Operator19/2
  DTC_Couter/2 -> Data Type Conversion1/1
  Logical Operator1/1 -> SR_Latch4/2
  Constant5/1 -> Logical Operator15/2
  Relay/1 -> SR_Latch3/1
  Logical Operator12/1 -> [VDDM_C3CCU1LCDFS_flg]  "VDDM_C3CCU1LCDFS_flg"
  Constant2/1 -> Switch1/1
  Switch5/1 -> Switch1/3, [VDDM_xxx_flg]
  Switch1/1 -> Test Detection Criteria/1
  [DTC_clear_request] -> Switch1/2
  [DTC_clear_request] -> DTC_Info/4
  Constant41/1 -> Test Detection Criteria/4
  [VDDM_C3CCU1LCDet_flg] -> DTC_Info/1
  [VDDM_C3CCU1LCCFS_flg] -> VDDM_C3CCU1LCCFS_flg/1, DTC_Info/3
  [VDDM_C3CCU1LCPass_flg] -> DTC_Info/2
  DTC_Info/1 -> VDDM_C3CCU1LCDTC_raw32/1  "VDDM_C3CCU1LCDTC_raw32"
  [task_time_s] -> Timer1/3
  [VPMM_PwrStaSW_enum] -> Equal2/1
  [VPMM_PwrStaSW_enum] -> Equal/1
  [VPMM_PowerSta_enum] -> Equal4/1
  Constant24/1 -> Switch4/1
  Demux/1 -> Unit Delay3/1
  [task_time_s] -> Test Detection Criteria/2
  Equal/1 -> Logical Operator2/2
  Logical Operator6/1 -> Timer1/1
  Constant19/1 -> Equal3/2
  Constant4/1 -> Equal4/2
  Logical Operator5/1 -> Switch6/2
  Switch3/1 -> Demux/1
  Constant21/1 -> Switch/3
  Constant3/1 -> Switch/1
  Constant22/1 -> Switch7/1
  [No_CAN3_BUS_OFF] -> Logical Operator2/1
  [VDDM_C3CCU1LCCFS_flg] -> Switch/2
  Constant28/1 -> Equal2/2
  Logical Operator2/1 -> Switch5/2
  [VDDM_C3CCU1LCPass_flg] -> Switch7/2
  [No_CAN3_BUS_OFF] -> Logical Operator5/1
  Constant40/1 -> Test Detection Criteria/3
  [VDDM_xxx_flg] -> SR_Latch1/2(reset)
  Constant26/1 -> Equal/2
  Switch/1 -> Goto19/1
  Equal2/1 -> Logical Operator5/2
  Constant18/1 -> Timer1/4
  Constant16/1 -> Switch6/3
  Timer1/1 -> Equal3/1
  Switch6/1 -> Timer1/2, Logical Operator6/1
  Constant27/1 -> Switch5/3
  Test Detection Criteria/1 -> [VDDM_C3CCU1LCDet_flg]  "VDDM_C3CCU1LCDet_flg"
  From19/1 -> Switch3/2
  Constant23/1 -> Switch7/3
  [VDDM_C3CCU1LCChk_flg] -> Switch5/1
  Switch7/1 -> [VDDM_C3CCU1LCDFSRls_flg]  "VDDM_C3CCU1LCDFSRls_flg"
  SR_Latch1/1(latched) -> [VDDM_C3CCU1LCPass_flg]  "VDDM_C3CCU1LCPass_flg"
  Logical Operator8/1 -> Switch4/2
  Equal3/1 -> SR_Latch1/1(set)
  [VDDM_C3CCU1LCChk_flg] -> Switch6/1
  [DTC_clear_request] -> Logical Operator8/2
  Constant25/1 -> Switch4/3
  Switch4/1 -> [VDDM_C3CCU1LCCFSRls_flg]  "VDDM_C3CCU1LCCFSRls_flg"
  Equal4/1 -> Logical Operator8/1
  No_CAN3_BUS_OFF/1 -> [No_CAN3_BUS_OFF]
  DTC_clear_request/1 -> [DTC_clear_request]
  task_time_s/1 -> [task_time_s]
  VDDM_C3CCU1LCChk_flg/1 -> [VDDM_C3CCU1LCChk_flg]
  VPMM_PwrStaSW_enum/1 -> [VPMM_PwrStaSW_enum]
  VPMM_PowerSta_enum/1 -> [VPMM_PowerSta_enum]

== system ddm/DDM/DDM/PMM/Comm err/VCU lost communication with CCU2 ==
  note: Diagnostics and Fault Handling
  note: Test Detection Criteria
  note: Release Condition During Failure Detection
  note: Fail Safe During Detection
  note: Release Condition After Failure Decision
  note: Test Pass Criteria
  note: Fail Safe After Decision
  task_time_s : Inport
  VPMM_PowerSta_enum : Inport  Port=2
  VPMM_PwrStaSW_enum : Inport  Port=3
  VDDM_C3CCU2LCChk_flg : Inport  Port=4
  No_CAN3_BUS_OFF : Inport  Port=5
  DTC_clear_request : Inport  Port=6
  Constant15 : Constant  Value=KDDM_C3CCU2LCCFSSW_flg
  Constant{3,16,22,24} (4 alike) : Constant  Value=TRUE
  Constant18 : Constant  Value=KDDM_C3CCU2LCPassTO_s
  Constant19 : Constant  Value=KDDM_C3CCU2LCPassTO_s
  Constant{2,21,23,25,27} (5 alike) : Constant  Value=FALSE
  Constant20 : Constant  Value=KDDM_C3CCU2LCDFSSW_flg
  Constant26 : Constant  Value=ENUM_PWRSTASW_OFF
  Constant28 : Constant  Value=ENUM_PWRSTASW_OFF
  Constant4 : Constant  Value=ENUM_POWERSTA_OFF
  Constant40 : Constant  Value=KDDM_C3CCU2LCDTC_cnt
  Constant41 : Constant  Value=KDDM_C3CCU2LCDetTO_s
  Constant46 : Constant  Value=KDDM_C3CCU2LCDetSW_flg
  Constant48 : Constant  Value=KDDM_C3CCU2LCDTC_cnt
  Constant5 : Constant  Value=KDDM_C3CCU2LCPassSW_flg
  DTC_Couter : hcu_lib/Basic_Blocks/DTC_Couter
  DTC_Info : hcu_lib/Basic_Blocks/DTC_Info
  Data Type Conversion1 : DataTypeConversion  OutDataTypeStr=uint8
  Demux : Demux  Commented=on  Outputs=5
  Equal : RelationalOperator  Operator=~=  OutDataTypeStr=boolean  RndMeth=Simplest
  Equal2 : RelationalOperator  Operator=~=  OutDataTypeStr=boolean  RndMeth=Simplest
  Equal3 : RelationalOperator  OutDataTypeStr=boolean  RndMeth=Simplest
  Equal4 : RelationalOperator  Operator===  OutDataTypeStr=boolean  RndMeth=Simplest
  From19 : From  Commented=on  GotoTag=VDDM_C3CCU2LCDFS_flg
  Goto19 : Goto  Commented=on  GotoTag=VDDM_EDriveSysErrVCUErr_flg
  Logical Operator1 : Logic  Operator=OR  AllPortsSameDT=off  OutDataTypeStr=boolean
  Logical Operator{2,5,12,15,18} (5 alike) : Logic  AllPortsSameDT=off  OutDataTypeStr=boolean
  Logical Operator19 : Logic  Inputs=3  AllPortsSameDT=off  OutDataTypeStr=boolean
  Logical Operator21 : Logic  Operator=OR  Inputs=3  AllPortsSameDT=off  OutDataTypeStr=boolean
  Logical Operator3 : Logic  Operator=OR  Inputs=3  AllPortsSameDT=off  OutDataTypeStr=boolean
  Logical Operator4 : Logic  Operator=NOT  AllPortsSameDT=off  OutDataTypeStr=boolean
  Logical Operator6 : Logic  Operator=NOT  AllPortsSameDT=off  OutDataTypeStr=boolean
  Logical Operator8 : Logic  Operator=OR  AllPortsSameDT=off  OutDataTypeStr=boolean
  Relay : Relay  OnSwitchValue=ONE_INT  OffSwitchValue=ZERO_INT
  SR_Latch1 : Subsystem  mask(SR_Latch){}
      mask help: SR latch function.
  SR_Latch3 : hcu_lib/Basic_Blocks/SR_Latch
  SR_Latch4 : hcu_lib/Basic_Blocks/SR_Latch
  Switch{,1,4..7} (6 alike) : Switch  Criteria=u2 ~= 0
  Switch3 : Switch  Commented=on  Criteria=u2 ~= 0
  Test Detection Criteria : hcu_lib/Basic_Blocks/Test Detection Criteria
  Timer1 : hcu_lib/Basic_Blocks/Timer
  Unit Delay3 : UnitDelay  Commented=on  SampleTime=-1  HasFrameUpgradeWarning=on
  VDDM_C3CCU2LCDTC_raw32 : Outport
  VDDM_C3CCU2LCCFS_flg : Outport  Port=2
  wires:
  Logical Operator15/1 -> DTC_Couter/2
  [DTC_clear_request] -> Logical Operator21/3
  [VDDM_C3CCU2LCDet_flg] -> Logical Operator19/1
  [DTC_clear_request] -> Logical Operator4/1
  Logical Operator1/1 -> SR_Latch4/2
  SR_Latch3/1 -> Logical Operator12/2
  Logical Operator3/1 -> Logical Operator15/1
  Logical Operator19/1 -> DTC_Couter/1
  Logical Operator4/1 -> Logical Operator19/3
  Constant5/1 -> Logical Operator15/2
  SR_Latch4/1 -> Logical Operator18/1
  Logical Operator21/1 -> SR_Latch3/2
  [VDDM_C3CCU2LCDTC_cnt] -> Relay/1
  DTC_Couter/2 -> Data Type Conversion1/1
  [VDDM_C3CCU2LCCFSRls_flg] -> Logical Operator1/1
  Constant20/1 -> Logical Operator12/1
  [VDDM_C3CCU2LCCFSRls_flg] -> Logical Operator3/2
  Relay/1 -> SR_Latch3/1
  [DTC_clear_request] -> Logical Operator3/3
  Logical Operator12/1 -> [VDDM_C3CCU2LCDFS_flg]  "VDDM_C3CCU2LCDFS_flg"
  Constant48/1 -> DTC_Couter/3
  [VDDM_C3CCU2LCDFSRls_flg] -> Logical Operator21/1
  [VDDM_C3CCU2LCPass_flg] -> Logical Operator3/1
  Logical Operator18/1 -> [VDDM_C3CCU2LCCFS_flg]  "VDDM_C3CCU2LCCFS_flg"
  Constant46/1 -> Logical Operator19/2
  DTC_Couter/1 -> SR_Latch4/1
  [VDDM_C3CCU2LCCFS_flg] -> Logical Operator21/2
  Data Type Conversion1/1 -> [VDDM_C3CCU2LCDTC_cnt]  "VDDM_C3CCU2LCDTC_cnt"
  Constant15/1 -> Logical Operator18/2
  [DTC_clear_request] -> Logical Operator1/2
  Constant2/1 -> Switch1/1
  Switch5/1 -> Switch1/3, [VDDM_xxx_flg]
  Switch1/1 -> Test Detection Criteria/1
  [DTC_clear_request] -> Switch1/2
  [DTC_clear_request] -> DTC_Info/4
  Constant41/1 -> Test Detection Criteria/4
  [VDDM_C3CCU2LCDet_flg] -> DTC_Info/1
  [VDDM_C3CCU2LCCFS_flg] -> VDDM_C3CCU2LCCFS_flg/1, DTC_Info/3
  [VDDM_C3CCU2LCPass_flg] -> DTC_Info/2
  DTC_Info/1 -> VDDM_C3CCU2LCDTC_raw32/1  "VDDM_C3CCU2LCDTC_raw32"
  [task_time_s] -> Timer1/3
  [VPMM_PwrStaSW_enum] -> Equal2/1
  [VPMM_PwrStaSW_enum] -> Equal/1
  [VPMM_PowerSta_enum] -> Equal4/1
  Logical Operator2/1 -> Switch5/2
  [VDDM_C3CCU2LCPass_flg] -> Switch7/2
  Logical Operator5/1 -> Switch6/2
  Constant27/1 -> Switch5/3
  Switch6/1 -> Timer1/2, Logical Operator6/1
  Timer1/1 -> Equal3/1
  Constant16/1 -> Switch6/3
  Constant18/1 -> Timer1/4
  From19/1 -> Switch3/2
  Test Detection Criteria/1 -> [VDDM_C3CCU2LCDet_flg]  "VDDM_C3CCU2LCDet_flg"
  Switch3/1 -> Demux/1
  Demux/1 -> Unit Delay3/1
  Constant21/1 -> Switch/3
  Constant4/1 -> Equal4/2
  [No_CAN3_BUS_OFF] -> Logical Operator2/1
  [task_time_s] -> Test Detection Criteria/2
  Constant19/1 -> Equal3/2
  Constant24/1 -> Switch4/1
  Logical Operator6/1 -> Timer1/1
  Equal/1 -> Logical Operator2/2
  [VDDM_C3CCU2LCCFS_flg] -> Switch/2
  Constant28/1 -> Equal2/2
  [VDDM_C3CCU2LCChk_flg] -> Switch5/1
  Constant22/1 -> Switch7/1
  Constant3/1 -> Switch/1
  Switch4/1 -> [VDDM_C3CCU2LCCFSRls_flg]  "VDDM_C3CCU2LCCFSRls_flg"
  Equal4/1 -> Logical Operator8/1
  Constant25/1 -> Switch4/3
  [DTC_clear_request] -> Logical Operator8/2
  [VDDM_C3CCU2LCChk_flg] -> Switch6/1
  Equal3/1 -> SR_Latch1/1(set)
  Logical Operator8/1 -> Switch4/2
  Switch7/1 -> [VDDM_C3CCU2LCDFSRls_flg]  "VDDM_C3CCU2LCDFSRls_flg"
  Constant23/1 -> Switch7/3
  SR_Latch1/1(latched) -> [VDDM_C3CCU2LCPass_flg]  "VDDM_C3CCU2LCPass_flg"
  [No_CAN3_BUS_OFF] -> Logical Operator5/1
  [VDDM_xxx_flg] -> SR_Latch1/2(reset)
  Constant40/1 -> Test Detection Criteria/3
  Equal2/1 -> Logical Operator5/2
  Constant26/1 -> Equal/2
  Switch/1 -> Goto19/1
  DTC_clear_request/1 -> [DTC_clear_request]
  No_CAN3_BUS_OFF/1 -> [No_CAN3_BUS_OFF]
  VPMM_PowerSta_enum/1 -> [VPMM_PowerSta_enum]
  VPMM_PwrStaSW_enum/1 -> [VPMM_PwrStaSW_enum]
  VDDM_C3CCU2LCChk_flg/1 -> [VDDM_C3CCU2LCChk_flg]
  task_time_s/1 -> [task_time_s]
